simulink model "yoyo"  (R2013b)
settings: Solver=ode45  StartTime=0.0  StopTime=10.0  RelTol=1e-3
values from neighbouring files (symbols this model uses):
  A = 1    [yoyo_model.m]    (also in yoyo_model_simulate.m; yoyo_model_testing_lqi.m)
  B = phi    [yoyo_model.m]    (also in yoyo_model_simulate.m; yoyo_model_testing_lqi.m = 1)
  C = 1    [yoyo_model.m]    (also in yoyo_model_simulate.m; yoyo_model_testing_lqi.m)
  const = psi/phi    [yoyo_model.m]    (also in yoyo_model_simulate.m; yoyo_model_testing_lqi.m = -100)
  D = 0    [yoyo_model.m]    (also in yoyo_model_simulate.m; yoyo_model_testing_lqi.m)
  H = 1    [yoyo_model.m]    (also in yoyo_model_simulate.m = -100; yoyo_model_testing_lqi.m)
  K = 1    [yoyo_model.m]    (also in yoyo_model_simulate.m = 0.001; yoyo_model_testing_lqi.m)
  yr = 0    [yoyo_model.m]    (also in yoyo_model_simulate.m; yoyo_model_testing_lqi.m)
libraries: simulink x1
settings Model: Creator=thomasesch  LastModifiedBy=thomasesch

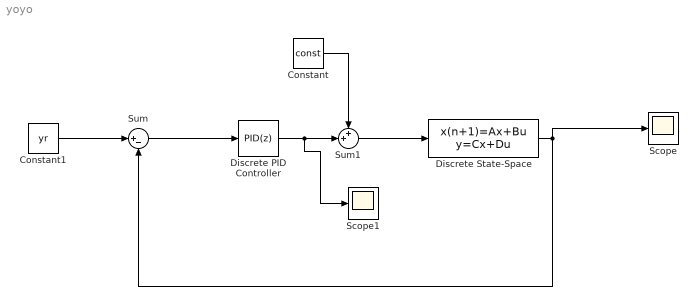
== system yoyo ==
  Constant : Constant  Value=const
  Constant1 : Constant  Value=yr
  Discrete PID Controller : simulink/Continuous/PID Controller  Controller=PID  TimeDomain=Discrete-time  SampleTime=1  IntegratorMethod=Forward Euler  FilterMethod=Forward Euler  Form=Parallel  P=-H  I=K  D=0  N=100  InitialConditionSource=internal  InitialConditionForIntegrator=0  InitialConditionForFilter=0  ExternalReset=none  LimitOutput=off  UpperSaturationLimit=inf  LowerSaturationLimit=-inf  LinearizeAsGain=off  AntiWindupMode=none  Kb=1  TrackingMode=off  Kt=1  PParamMin=[]  PParamMax=[]  IParamMin=[]  IParamMax=[]  DParamMin=[]  DParamMax=[]  NParamMin=[]  NParamMax=[]  KbParamMin=[]  KbParamMax=[]  KtParamMin=[]  KtParamMax=[]  POutMin=[]  POutMax=[]  IOutMin=[]  IOutMax=[]  DOutMin=[]  DOutMax=[]  NOutMin=[]  NOutMax=[]  KbOutMin=[]  KbOutMax=[]  KtOutMin=[]  KtOutMax=[]  IntegratorOutMin=[]  IntegratorOutMax=[]  FilterOutMin=[]  FilterOutMax=[]  SumOutMin=[]  SumOutMax=[]  SumI1OutMin=[]  SumI1OutMax=[]  SumI2OutMin=[]  SumI2OutMax=[]  SumI3OutMin=[]  SumI3OutMax=[]  SumDOutMin=[]  SumDOutMax=[]  SaturationOutMin=[]  SaturationOutMax=[]  IntegratorContinuousStateAttributes=''  IntegratorStateMustResolveToSignalObject=off  IntegratorRTWStateStorageClass=Auto  FilterContinuousStateAttributes=''  FilterStateMustResolveToSignalObject=off  FilterRTWStateStorageClass=Auto
  Discrete State-Space : DiscreteStateSpace  A=A  B=B  C=C  D=D
  Scope : Scope
  Scope1 : Scope
  Sum : Sum  Inputs=|+-
  Sum1 : Sum  Inputs=++|
  wires:
  Discrete State-Space/1 -> Sum/2, Scope/1
  Sum/1 -> Discrete PID Controller/1
  Discrete PID Controller/1 -> Scope1/1, Sum1/2
  Sum1/1 -> Discrete State-Space/1
  Constant/1 -> Sum1/1
  Constant1/1 -> Sum/1
